simulink library "actuators_lib"  (R2016b)
settings: Solver=ode45  StartTime=0.0  StopTime=10.0  RelTol=1e-3  EnableMultiTasking=on
undefined symbols (not defined in the file or in its folder): current_RW_RPM, magnetic_dipole, magnetorquer_pwrstate, MT_on, MT_power_OK, RW_pwrstate, torque
undefined symbols (not defined in the file): sim_params
libraries: simulink x3, bus_stubs_template x2, RW_assembly_simple_lib x1
settings Model: Creator=bbarz_000  LastModifiedBy=taylorreynolds
settings DataIOCC: LimitDataPoints=on
settings OptimizationCC: LifeSpan=inf
settings DebuggingCC: AllowSymbolicDim=off  SFUnexpectedBacktrackingDiag=warning  SFNoUnconditionalDefaultTransitionDiag=warning  SFExecutionAtInitializationDiag=none
settings GRTTargetCC: TargetLangStandard=C89/C90 (ANSI)  GeneratePreprocessorConditionals=Disable all
settings ConfigComp: CovMetricSettings=dw  CovHtmlReporting=on  CovSaveCumulativeToWorkspaceVar=on  CovSaveSingleToWorkspaceVar=on  CovExternalEMLEnable=off

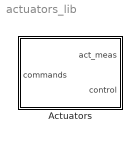
== system actuators_lib ==
  Actuators : Subsystem

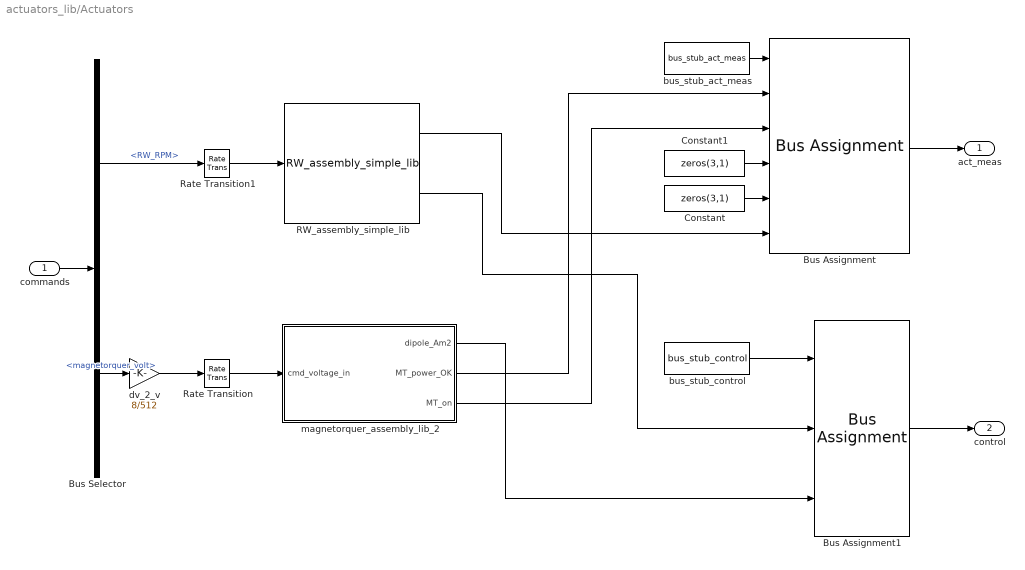
== system actuators_lib/Actuators ==
  commands : Inport  OutDataTypeStr=Bus: commands
  Bus Assignment : BusAssignment  AssignedSignals=MT_power_OK,MT_on,RW_pwrstate,magnetorquer_pwrstate,current_RW_RPM
  Bus Assignment1 : BusAssignment  AssignedSignals=torque,magnetic_dipole
  Bus Selector : BusSelector  OutputSignals=RW_RPM,magnetorquer_volt
  Constant : Constant  Value=zeros(3,1)
  Constant1 : Constant  Value=zeros(3,1)
  RW_assembly_simple_lib : RW_assembly_simple_lib/RW_assembly_simple_lib  natural_frequency=sim_params.actuators.reaction_wheel.natural_freq  damping_ratio=sim_params.actuators.reaction_wheel.damping  max_rate=sim_params.actuators.reaction_wheel.rate_limit
  Rate Transition : RateTransition  OutPortSampleTime=1/20
  Rate Transition1 : RateTransition  OutPortSampleTime=1/20
  bus_stub_act_meas : bus_stubs_template/bus_stub_act_meas
  bus_stub_control : bus_stubs_template/bus_stub_control
  dv_2_v : Gain  Gain=8/512
  magnetorquer_assembly_lib_2 : Subsystem
  act_meas : Outport
  control : Outport  Port=2
  wires:
  Rate Transition1/1 -> RW_assembly_simple_lib/1
  Rate Transition/1 -> magnetorquer_assembly_lib_2/1(cmd_voltage_in)
  dv_2_v/1 -> Rate Transition/1
  commands/1 -> Bus Selector/1
  Bus Assignment/1 -> act_meas/1
  bus_stub_act_meas/1 -> Bus Assignment/1
  bus_stub_control/1 -> Bus Assignment1/1
  Bus Assignment1/1 -> control/1
  Bus Selector/1 -> Rate Transition1/1  "<RW_RPM>"
  Bus Selector/2 -> dv_2_v/1  "<magnetorquer_volt>"
  RW_assembly_simple_lib/2 -> Bus Assignment1/2
  magnetorquer_assembly_lib_2/1(dipole_Am2) -> Bus Assignment1/3
  magnetorquer_assembly_lib_2/2(MT_power_OK) -> Bus Assignment/2
  magnetorquer_assembly_lib_2/3(MT_on) -> Bus Assignment/3
  RW_assembly_simple_lib/1 -> Bus Assignment/6
  Constant/1 -> Bus Assignment/5
  Constant1/1 -> Bus Assignment/4

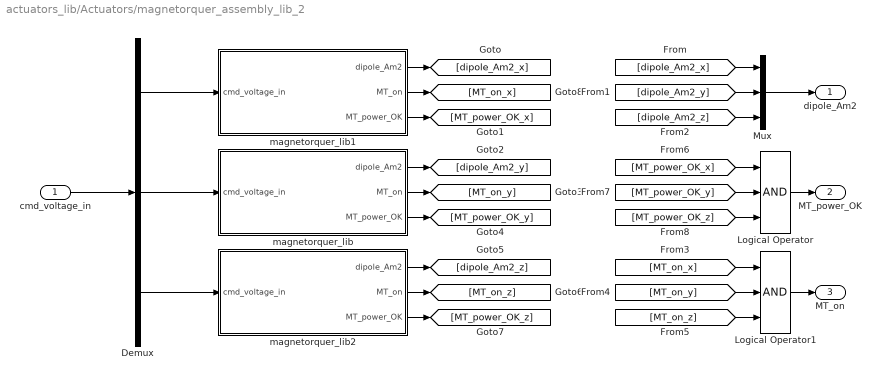
== system actuators_lib/Actuators/magnetorquer_assembly_lib_2 ==
  cmd_voltage_in : Inport
  Demux : Demux  Outputs=3
  Logical Operator : Logic  Inputs=3  AllPortsSameDT=off  OutDataTypeStr=boolean
  Logical Operator1 : Logic  Inputs=3  AllPortsSameDT=off  OutDataTypeStr=boolean
  Mux : Mux  Inputs=3
  magnetorquer_lib : Subsystem  mask{voltage_to_dipole=0.25*sim_params.actuators.magnetorquer.max_dipole_y, upperbound=sim_params.actuators.magnetorquer.max_dipole_y, lowerbound=-sim_params.actuators.magnetorquer.max_dipole_y}
      mask prompts: voltage_to_dipole "Simulink:blkprm_prompts:GainGain"; upperbound "Simulink:masks:UpperBound_MP"; lowerbound "Simulink:masks:LowerBound_MP"
      mask TypeOptions voltage_to_dipole: Gain/Gain
      mask TypeOptions upperbound:
      | Check
      | Static Range/max
      mask TypeOptions lowerbound:
      | Check
      | Static Range/min
  magnetorquer_lib1 : Subsystem  mask{voltage_to_dipole=0.25*sim_params.actuators.magnetorquer.max_dipole_x, upperbound=sim_params.actuators.magnetorquer.max_dipole_x, lowerbound=-sim_params.actuators.magnetorquer.max_dipole_x}
      mask prompts: voltage_to_dipole "Simulink:blkprm_prompts:GainGain"; upperbound "Simulink:masks:UpperBound_MP"; lowerbound "Simulink:masks:LowerBound_MP"
      mask TypeOptions voltage_to_dipole: Gain/Gain
      mask TypeOptions upperbound:
      | Check
      | Static Range/max
      mask TypeOptions lowerbound:
      | Check
      | Static Range/min
  magnetorquer_lib2 : Subsystem  mask{voltage_to_dipole=0.25*sim_params.actuators.magnetorquer.max_dipole_z, upperbound=sim_params.actuators.magnetorquer.max_dipole_z, lowerbound=-sim_params.actuators.magnetorquer.max_dipole_z}
      mask prompts: voltage_to_dipole "Simulink:blkprm_prompts:GainGain"; upperbound "Simulink:masks:UpperBound_MP"; lowerbound "Simulink:masks:LowerBound_MP"
      mask TypeOptions voltage_to_dipole: Gain/Gain
      mask TypeOptions upperbound:
      | Check
      | Static Range/max
      mask TypeOptions lowerbound:
      | Check
      | Static Range/min
  dipole_Am2 : Outport
  MT_power_OK : Outport  Port=2
  MT_on : Outport  Port=3
  wires:
  cmd_voltage_in/1 -> Demux/1
  Demux/3 -> magnetorquer_lib2/1(cmd_voltage_in)
  Demux/1 -> magnetorquer_lib1/1(cmd_voltage_in)
  Demux/2 -> magnetorquer_lib/1(cmd_voltage_in)
  magnetorquer_lib1/1(dipole_Am2) -> [dipole_Am2_x]
  magnetorquer_lib2/3(MT_power_OK) -> [MT_power_OK_z]
  magnetorquer_lib2/2(MT_on) -> [MT_on_z]
  magnetorquer_lib2/1(dipole_Am2) -> [dipole_Am2_z]
  magnetorquer_lib/3(MT_power_OK) -> [MT_power_OK_y]
  magnetorquer_lib/2(MT_on) -> [MT_on_y]
  magnetorquer_lib/1(dipole_Am2) -> [dipole_Am2_y]
  magnetorquer_lib1/3(MT_power_OK) -> [MT_power_OK_x]
  magnetorquer_lib1/2(MT_on) -> [MT_on_x]
  Mux/1 -> dipole_Am2/1
  [dipole_Am2_x] -> Mux/1
  [dipole_Am2_y] -> Mux/2
  [dipole_Am2_z] -> Mux/3
  [MT_on_x] -> Logical Operator1/1
  [MT_on_y] -> Logical Operator1/2
  [MT_on_z] -> Logical Operator1/3
  [MT_power_OK_x] -> Logical Operator/1
  [MT_power_OK_y] -> Logical Operator/2
  [MT_power_OK_z] -> Logical Operator/3
  Logical Operator/1 -> MT_power_OK/1
  Logical Operator1/1 -> MT_on/1

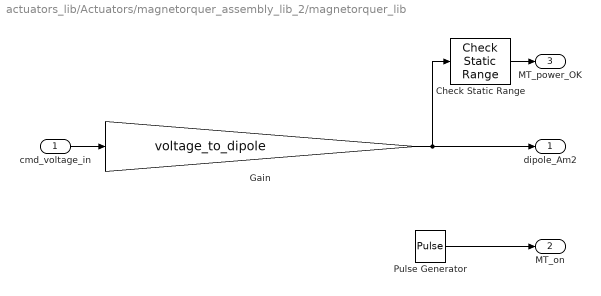
== system actuators_lib/Actuators/magnetorquer_assembly_lib_2/magnetorquer_lib ==
  cmd_voltage_in : Inport
  Check Static Range : simulink/Model Verification/Check  Static Range  Description=lowerbound <= u <= upperbound  max=upperbound  max_included=on  min=lowerbound  min_included=on  enabled=on  stopWhenAssertionFail=off  export=on  icon=graphic
  Gain : Gain  Gain=voltage_to_dipole
  Pulse Generator : DiscretePulseGenerator  PulseType=Time based  Period=1  PulseWidth=fsw_params.actuators.magnetorquer.actuation_time_pct
  dipole_Am2 : Outport
  MT_on : Outport  Port=2
  MT_power_OK : Outport  Port=3
  wires:
  cmd_voltage_in/1 -> Gain/1
  Gain/1 -> Check Static Range/1, dipole_Am2/1
  Pulse Generator/1 -> MT_on/1
  Check Static Range/1 -> MT_power_OK/1

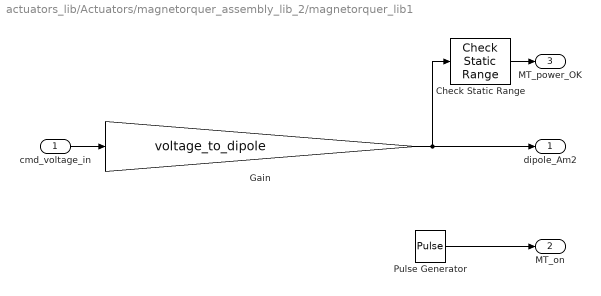
== system actuators_lib/Actuators/magnetorquer_assembly_lib_2/magnetorquer_lib1 ==
  cmd_voltage_in : Inport
  Check Static Range : simulink/Model Verification/Check  Static Range  Description=lowerbound <= u <= upperbound  max=upperbound  max_included=on  min=lowerbound  min_included=on  enabled=on  stopWhenAssertionFail=off  export=on  icon=graphic
  Gain : Gain  Gain=voltage_to_dipole
  Pulse Generator : DiscretePulseGenerator  PulseType=Time based  Period=1  PulseWidth=fsw_params.actuators.magnetorquer.actuation_time_pct
  dipole_Am2 : Outport
  MT_on : Outport  Port=2
  MT_power_OK : Outport  Port=3
  wires:
  cmd_voltage_in/1 -> Gain/1
  Gain/1 -> Check Static Range/1, dipole_Am2/1
  Pulse Generator/1 -> MT_on/1
  Check Static Range/1 -> MT_power_OK/1

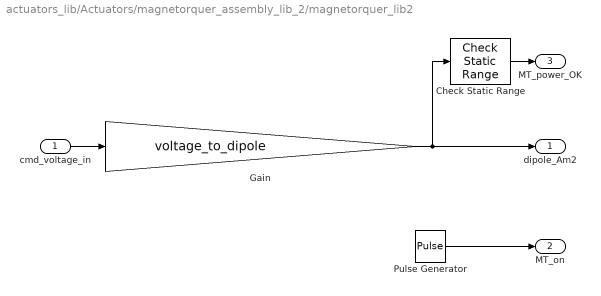
== system actuators_lib/Actuators/magnetorquer_assembly_lib_2/magnetorquer_lib2 ==
  cmd_voltage_in : Inport
  Check Static Range : simulink/Model Verification/Check  Static Range  Description=lowerbound <= u <= upperbound  max=upperbound  max_included=on  min=lowerbound  min_included=on  enabled=on  stopWhenAssertionFail=off  export=on  icon=graphic
  Gain : Gain  Gain=voltage_to_dipole
  Pulse Generator : DiscretePulseGenerator  PulseType=Time based  Period=1  PulseWidth=fsw_params.actuators.magnetorquer.actuation_time_pct
  dipole_Am2 : Outport
  MT_on : Outport  Port=2
  MT_power_OK : Outport  Port=3
  wires:
  cmd_voltage_in/1 -> Gain/1
  Gain/1 -> Check Static Range/1, dipole_Am2/1
  Pulse Generator/1 -> MT_on/1
  Check Static Range/1 -> MT_power_OK/1
